simulink model "ir_info_sim"  (R2016a)
settings: Solver=VariableStepAuto  StartTime=0.0  StopTime=10.0  RelTol=1e-3
libraries: simulink x7
settings Model: Creator=maximilian  LastModifiedBy=marlene

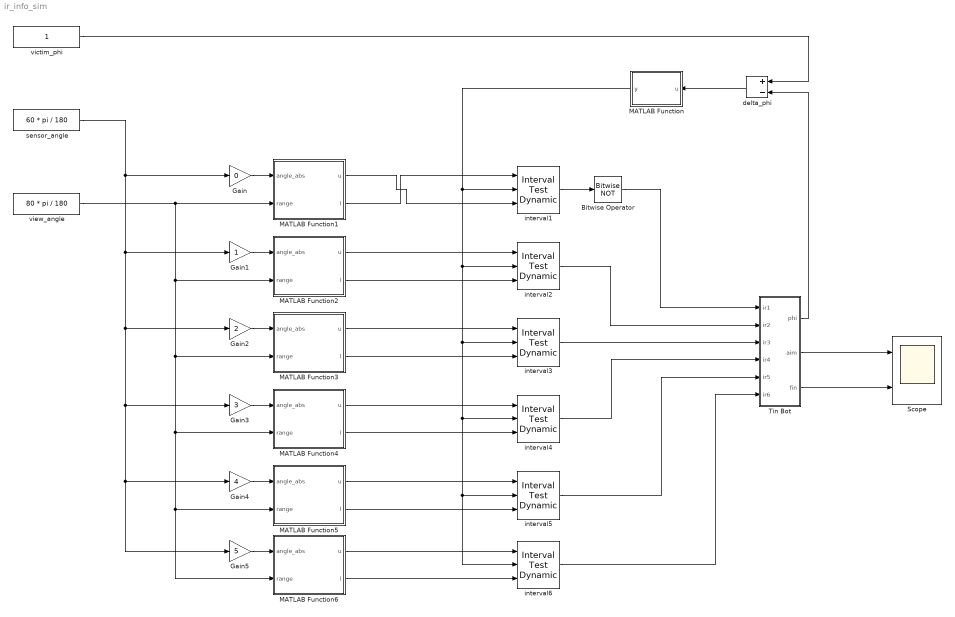
== system ir_info_sim ==
  Bitwise Operator : simulink/Logic and Bit Operations/Bitwise Operator  logicop=NOT  UseBitMask=off  BitMask=bin2dec('11011001')  BitMaskRealWorld=Stored Integer
  Gain : Gain  Gain=0
  Gain1 : Gain
  Gain2 : Gain  Gain=2
  Gain3 : Gain  Gain=3
  Gain4 : Gain  Gain=4
  Gain5 : Gain  Gain=5
  MATLAB Function : MATLAB Function  TreatAsAtomicUnit=on
  MATLAB Function1 : MATLAB Function  TreatAsAtomicUnit=on
  MATLAB Function2 : MATLAB Function  TreatAsAtomicUnit=on
  MATLAB Function3 : MATLAB Function  TreatAsAtomicUnit=on
  MATLAB Function4 : MATLAB Function  TreatAsAtomicUnit=on
  MATLAB Function5 : MATLAB Function  TreatAsAtomicUnit=on
  MATLAB Function6 : MATLAB Function  TreatAsAtomicUnit=on
  Scope : Scope  NumInputPorts=2
  Tin Bot : Subsystem
  delta_phi : Sum  Inputs=+-
  interval{1..6} (6 alike) : simulink/Logic and Bit Operations/Interval Test Dynamic  IntervalClosedRight=on  IntervalClosedLeft=on  OutDataTypeStr=boolean
  sensor_angle : Constant  Value=60 * pi / 180
  victim_phi : Constant
  view_angle : Constant  Value=80 * pi / 180
  wires:
  victim_phi/1 -> delta_phi/1
  Tin Bot/1(phi) -> delta_phi/2
  delta_phi/1 -> MATLAB Function/1(u)
  interval1/1 -> Bitwise Operator/1
  interval2/1 -> Tin Bot/2(ir2)
  interval3/1 -> Tin Bot/3(ir3)
  interval4/1 -> Tin Bot/4(ir4)
  interval5/1 -> Tin Bot/5(ir5)
  interval6/1 -> Tin Bot/6(ir6)
  MATLAB Function/1(y) -> interval6/2, interval5/2, interval4/2, interval3/2, interval2/2, interval1/2
  MATLAB Function1/2(l) -> interval1/1
  MATLAB Function6/1(u) -> interval6/1
  MATLAB Function6/2(l) -> interval6/3
  MATLAB Function5/1(u) -> interval5/1
  MATLAB Function5/2(l) -> interval5/3
  MATLAB Function4/1(u) -> interval4/1
  MATLAB Function4/2(l) -> interval4/3
  MATLAB Function3/1(u) -> interval3/1
  MATLAB Function3/2(l) -> interval3/3
  MATLAB Function2/1(u) -> interval2/1
  MATLAB Function2/2(l) -> interval2/3
  Gain/1 -> MATLAB Function1/1(angle_abs)
  Gain1/1 -> MATLAB Function2/1(angle_abs)
  Gain2/1 -> MATLAB Function3/1(angle_abs)
  Gain3/1 -> MATLAB Function4/1(angle_abs)
  Gain4/1 -> MATLAB Function5/1(angle_abs)
  Gain5/1 -> MATLAB Function6/1(angle_abs)
  sensor_angle/1 -> Gain5/1, Gain4/1, Gain3/1, Gain2/1, Gain1/1, Gain/1
  view_angle/1 -> MATLAB Function6/2(range), MATLAB Function5/2(range), MATLAB Function4/2(range), MATLAB Function3/2(range), MATLAB Function2/2(range), MATLAB Function1/2(range)
  Bitwise Operator/1 -> Tin Bot/1(ir1)
  MATLAB Function1/1(u) -> interval1/3
  Tin Bot/2(aim) -> Scope/1
  Tin Bot/3(fin) -> Scope/2

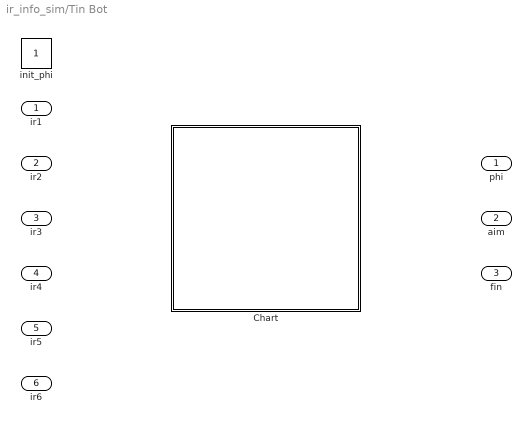
== system ir_info_sim/Tin Bot ==
  ir1 : Inport
  ir2 : Inport  Port=2
  ir3 : Inport  Port=3
  ir4 : Inport  Port=4
  ir5 : Inport  Port=5
  ir6 : Inport  Port=6
  Chart : Stateflow chart  TreatAsAtomicUnit=on
  init_phi : Constant
  phi : Outport
  aim : Outport  Port=2
  fin : Outport  Port=3

== matlab function ir_info_sim/MATLAB Function1 ==
  data: angle_abs input; u output; range input; l output
function [u, l] = fnc(angle_abs, range)
    u = mod(angle_abs+range/2, 2*pi);
    l = mod(angle_abs-range/2, 2*pi);
end

== matlab function ir_info_sim/MATLAB Function ==
  data: u input; y output
function y = mod(u)
    y = mod(u, 2*pi);
end

== matlab function ir_info_sim/MATLAB Function2 ==
  data: angle_abs input; u output; range input; l output
function [u, l] = fnc(angle_abs, range)
    u = mod(angle_abs+range/2, 2*pi);
    l = mod(angle_abs-range/2, 2*pi);
end

== matlab function ir_info_sim/MATLAB Function3 ==
  data: angle_abs input; u output; range input; l output
function [u, l] = fnc(angle_abs, range)
    u = mod(angle_abs+range/2, 2*pi);
    l = mod(angle_abs-range/2, 2*pi);
end

== matlab function ir_info_sim/MATLAB Function4 ==
  data: angle_abs input; u output; range input; l output
function [u, l] = fnc(angle_abs, range)
    u = mod(angle_abs+range/2, 2*pi);
    l = mod(angle_abs-range/2, 2*pi);
end

== matlab function ir_info_sim/MATLAB Function5 ==
  data: angle_abs input; u output; range input; l output
function [u, l] = fnc(angle_abs, range)
    u = mod(angle_abs+range/2, 2*pi);
    l = mod(angle_abs-range/2, 2*pi);
end

== matlab function ir_info_sim/MATLAB Function6 ==
  data: angle_abs input; u output; range input; l output
function [u, l] = fnc(angle_abs, range)
    u = mod(angle_abs+range/2, 2*pi);
    l = mod(angle_abs-range/2, 2*pi);
end

== stateflow chart ir_info_sim/Tin Bot/Chart ==
